simulink model "imucalibration"  (Simulink 7.5)
settings: Solver=ode3  StartTime=0.0  StopTime=inf  FixedStep=.05  RelTol=1e-3
undefined symbols (not defined in the file or in its folder): CR, serial
libraries: instrumentlib x2, realtime_pacer_lib x1
settings Model: Creator=TCA  LastModifiedBy=meuser
settings OptimizationCC: InitFltsAndDblsToZero=on
settings DebuggingCC: StrictBusMsg=Warning

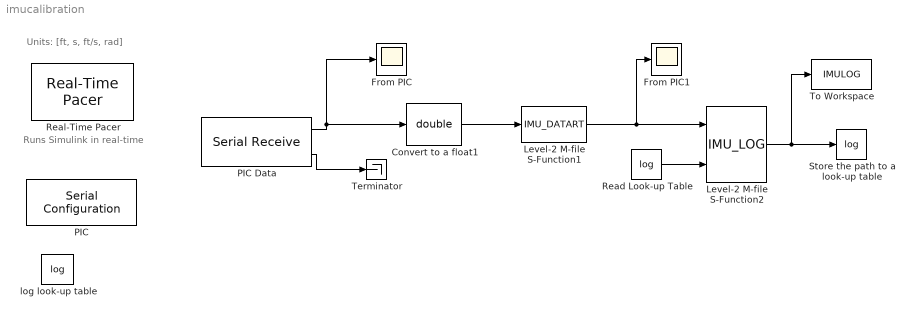
== system imucalibration ==
  note: Runs Simulink
      |  in real-time
  note: Units: [ft, s, ft/s, rad]
  Convert to a float1 : DataTypeConversion  OutDataTypeMode=double  OutDataTypeStr=double  SaturateOnIntegerOverflow=on  RndMeth=Zero
  From PIC : Scope
      settings: TimeRange=10  YMin=0  YMax=180
  From PIC1 : Scope
      settings: TimeRange=10  YMin=375  YMax=800
  Level-2 M-file S-Function1 : M-S-Function  FunctionName=IMU_DATART  Parameters=1
  Level-2 M-file S-Function2 : M-S-Function  FunctionName=IMU_LOG  Parameters=1
  PIC : instrumentlib/Serial Configuration  Priority=-200000  DialogController=instrumentcreatedialog  DialogControllerArgs=DataTag0  ComPortMenu=COM5  ComPort=COM5  ObjConstructor=serial('COM5');  BaudRate=9600  DataBits=8  Parity=none  StopBits=1  FlowControl=none  Timeout=10  ByteOrder=LittleEndian
  PIC Data : instrumentlib/Serial Receive  DialogController=instrumentcreatedialog  DialogControllerArgs=DataTag1  ComPortMenu=COM5  ComPort=COM5  ObjConstructor=serial('COM5');  Terminator=CR ('\r')  DataSize="[1  16]"  DataType=uint8  EnableBlockingMode=off  ActionDataUnavailable=Output last received value  CustomValue=0  SampleTime=.05
  Read Look-up Table : DataStoreRead  DataStoreName=log  SampleTime=0
  Real-Time Pacer : realtime_pacer_lib/Real-Time Pacer  simTimePerRealTime=1
  Store the path to a look-up table : DataStoreWrite  DataStoreName=log  SampleTime=-1
  Terminator : Terminator
  To Workspace : ToWorkspace  VariableName=IMULOG  SampleTime=-1  SaveFormat=Array
  log look-up table : DataStoreMemory  DataStoreName=log  ReadBeforeWriteMsg=warning  WriteAfterWriteMsg=warning  WriteAfterReadMsg=warning  InitialValue=zeros(2001, 6)  VectorParams1D=off
  wires:
  Convert to a float1/1 -> Level-2 M-file S-Function1/1
  PIC Data/1 -> From PIC/1, Convert to a float1/1
  Level-2 M-file S-Function1/1 -> From PIC1/1, Level-2 M-file S-Function2/1
  PIC Data/2 -> Terminator/1
  Read Look-up Table/1 -> Level-2 M-file S-Function2/2
  Level-2 M-file S-Function2/1 -> Store the path to a look-up table/1, To Workspace/1
